simulink model "Valve_SimScape"  (R2023a)
settings: Solver=VariableStepAuto  StartTime=0.0  StopTime=8  RelTol=1e-3  AbsTol=1e-3
libraries: fl_lib x5, nesl_utility x5, SimscapeFluids_lib x1, simulink x1
settings Model: Creator=xuluyu  LastModifiedBy=xuluyu
settings SolverCC: AutoScaleAbsTol=off  AlgebraicLoopSolver=TrustRegion  MaxZcPerStep=1
settings DebuggingCC: UnconnectedInputMsg=warning  UnconnectedOutputMsg=warning  UnconnectedLineMsg=warning  SymbolicDimsDataTypeCodeGenerationDiagnostic=none
settings ModelReferenceCC: EnableRefExpFcnMdlSchedulingChecks=on
settings SFSimCC: CustomCodeUndefinedFunction=UseInterfaceOnly
settings RTWCC: DLArmComputeVersion=19.05
settings SimscapeCC: SimscapeLogType=all  SimscapeLogSimulationStatistics=on  SimscapeLogOpenViewer=on  SimscapeLogLimitData=off  SimscapeLogDataHistory=10000

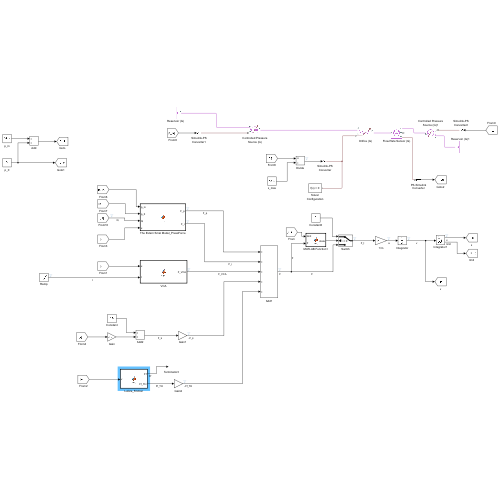
[thumbnail: Simulink's stored preview of the top-level diagram]
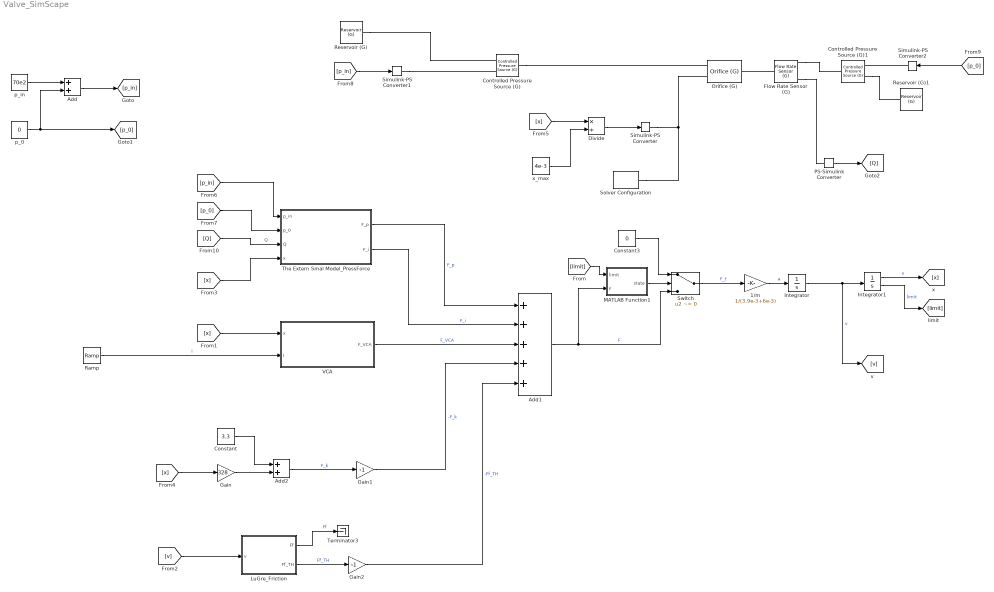
== system Valve_SimScape ==
  1/m : Gain  Gain=1/(3.9e-3+6e-3)
  Add : Sum
  Add1 : Sum  Inputs=+++++
  Add2 : Sum
  Constant : Constant  Value=3.3
  Constant3 : Constant  Value=0
  Controlled Pressure Source (G) : fl_lib/Gas/Sources/Controlled Pressure Source (G)  power_spec=foundation.enum.power_spec.isentropic  area_A=0.01 m^2  area_B=0.01 m^2
      settings: InternalSimscapePortConfiguration="{\"Bottom\":[],\"Left\":[{\"id\":\"A\",\"label\":\"A\",\"type\":\"foundation.gas.gas\"},{\"id\":\"P\",\"label\":\"P\",\"type\":\"input\"}],\"Right\":[{\"id\":\"B\",\"label\":\"B\",\"type\":\"foundation.gas.gas\"}],\"Top\":[]}"
  Controlled Pressure Source (G)1 : fl_lib/Gas/Sources/Controlled Pressure Source (G)  power_spec=foundation.enum.power_spec.isentropic  area_A=0.01 m^2  area_B=0.01 m^2
      settings: InternalSimscapePortConfiguration="{\"Bottom\":[],\"Left\":[{\"id\":\"A\",\"label\":\"A\",\"type\":\"foundation.gas.gas\"},{\"id\":\"P\",\"label\":\"P\",\"type\":\"input\"}],\"Right\":[{\"id\":\"B\",\"label\":\"B\",\"type\":\"foundation.gas.gas\"}],\"Top\":[]}"
  Divide : Product  Inputs=*/
  Flow Rate Sensor (G) : fl_lib/Gas/Sensors/Flow Rate Sensor (G)  mass_flow_measure=true  volumetric_flow_measure=true  volumetric_flow_conditions=foundation.enum.volumetric_flow_conditions.actual  p_std=0.101325 MPa  T_std=20 degC  energy_flow_measure=false
      settings: InternalSimscapePortConfiguration="{\"Bottom\":[],\"Left\":[{\"id\":\"A\",\"label\":\"A\",\"type\":\"foundation.gas.gas\"}],\"Right\":[{\"id\":\"B\",\"label\":\"B\",\"type\":\"foundation.gas.gas\"},{\"id\":\"M\",\"label\":\"M\",\"type\":\"output\"},{\"id\":\"V\",\"label\":\"V\",\"type\":\"output\"}],\"Top\":[]}"
  Gain : Gain  Gain=328
  Gain1 : Gain  Gain=-1
  Gain2 : Gain  Gain=-1
  Integrator : Integrator
  Integrator1 : Integrator  InitialCondition=1e-8  LimitOutput=on  UpperSaturationLimit=4e-3  LowerSaturationLimit=1e-8  ShowSaturationPort=on  ContinuousStateAttributes='x'
  LuGre_Friction : MATLAB Function  TreatAsAtomicUnit=on
  MATLAB Function1 : MATLAB Function  TreatAsAtomicUnit=on
  Orifice (G) : SimscapeFluids_lib/Gas/Valves & Orifices/Orifice (G)  orifice_type=foundation.enum.constant_variable.variable  orifice_parameterization=fluids.gas.valves_orifices.enum.OrificeParameterization.Cv  opening_characteristic=fluids.gas.valves_orifices.enum.OpeningCharacteristics.Tabulated  Cv_constant=4  Cv_max=4  L_Cv_TLU=Open_vector  Cv_TLU=Cv_valve  xT_Cv=0.7  Kv_constant=3.6  Kv_max=3.6  L_Kv_TLU=0 : 0.2 : 1  Kv_TLU=[1e-06, .72, 1.44, 2.16, 2.88, 3.6]  xT_Kv=0.7  C_constant=12 l/(bar*s)  B_crit_constant=0.3  C_max=12 l/(bar*s)  B_crit_linear=0.3  L_C_TLU=0 : 0.2 : 1  C_TLU=[1e-05, 2.4, 4.8, 7.2, 9.6, 12] l/(bar*s)  B_crit_TLU=0.3 * ones(1, 6)  m=0.5  T_ref_C=293.15 K  rho_ref_C=1.185 kg/m^3  orifice_area_constant=1e-4 m^2  orifice_area_max=1e-4 m^2  L_orifice_area_TLU=0 : 0.2 : 1  orifice_area_TLU=[1e-10, 2e-05, 4e-05, 6e-05, 8e-05, .0001] m^2  Cd=0.64  leakage_fraction=1e-6  smoothing_factor=0.01  B_lam=0.999  area=0.01 m^2
      settings: InternalSimscapePortConfiguration="{\"Bottom\":[],\"Left\":[{\"id\":\"A\",\"label\":\"A\",\"type\":\"foundation.gas.gas\"},{\"id\":\"L\",\"label\":\"L\",\"type\":\"input\"}],\"Right\":[{\"id\":\"B\",\"label\":\"B\",\"type\":\"foundation.gas.gas\"}],\"Top\":[]}"
  PS-Simulink Converter : nesl_utility/PS-Simulink Converter  PhysicalDomain=network_engine_domain  SubClassName=ps_output  LeftPortType=input  RightPortType=output  PseudoPeriodic=off  Frequencies=[]  VectorFormat=inherit  Unit=inherit  AffineConversion=off
  Ramp : simulink/Sources/Ramp  slope=1/5  start=1  InitialOutput=0
  Reservoir (G) : fl_lib/Gas/Elements/Reservoir (G)  pressure_spec=foundation.enum.pressure_spec.atmospheric  reservoir_pressure=0.101325 MPa  reservoir_temperature=293.15 K  area_A=0.01 m^2
  Reservoir (G)1 : fl_lib/Gas/Elements/Reservoir (G)  pressure_spec=foundation.enum.pressure_spec.atmospheric  reservoir_pressure=0.101325 MPa  reservoir_temperature=293.15 K  area_A=0.01 m^2
  Simulink-PS Converter : nesl_utility/Simulink-PS Converter  PhysicalDomain=network_engine_domain  SubClassName=ps_input  LeftPortType=input  RightPortType=output  PseudoPeriodic=off  Frequencies=[]  NoiseDistribution=none  NoiseParameters=[]  Unit=1  AffineConversion=off  FilteringAndDerivatives=provide  SimscapeFilterOrder=1  InputFilterTimeConstant=0.001  UdotUserProvided=0
  Simulink-PS Converter1 : nesl_utility/Simulink-PS Converter  PhysicalDomain=network_engine_domain  SubClassName=ps_input  LeftPortType=input  RightPortType=output  PseudoPeriodic=off  Frequencies=[]  NoiseDistribution=none  NoiseParameters=[]  Unit=Pa  AffineConversion=off  FilteringAndDerivatives=provide  SimscapeFilterOrder=1  InputFilterTimeConstant=0.001  UdotUserProvided=0
  Simulink-PS Converter2 : nesl_utility/Simulink-PS Converter  PhysicalDomain=network_engine_domain  SubClassName=ps_input  LeftPortType=input  RightPortType=output  PseudoPeriodic=off  Frequencies=[]  NoiseDistribution=none  NoiseParameters=[]  Unit=Pa  AffineConversion=off  FilteringAndDerivatives=provide  SimscapeFilterOrder=1  InputFilterTimeConstant=0.001  UdotUserProvided=0
  Solver Configuration : nesl_utility/Solver Configuration  PhysicalDomain=network_engine_domain  SubClassName=solver  LeftPortType=input  RightPortType=generic  Tones=[]  Harmonics=[]  SimulateNoise=off  Profile=off  UseLocalSampling=off  EnableSwitchedLinearOptims=on  FrequencyDomain=off  UseCCode=off  RelTol=0.001  AbsTol=1e-06  MinStep=1e-09  ToWorkspace=off  RevertToSquareIcSolve=off  NumHomotopyIterations=100  PhasorMode=off  PhasorModeNumHarmonics=1  ConsistencySolver=NEWTON_XTOL_AFTER_FTOL  IndexReductionMethod=DerivativeReplacement  DoDC=off  ResidualTolerance=1e-09  ConsistencyTolSource=GLOBAL  ConsistencyAbsTol=0.001  ConsistencyRelTol=0.001  ConsistencyTolFactor=0.001  UseLocalSolver=off  LocalSolverChoice=NE_BACKWARD_EULER_ADVANCER  ResolveIndetEquations=on  FunctionEvalNumThread=1  LocalSolverSampleTime=0.001  DoFixedCost=off  MaxNonlinIter=3  MaxModeIter=2  ComputeImpulses=off  ImpulseIterations=2  LinearAlgebra=auto  LinearAlgebraNumThread=0  EquationFormulation=NE_TIME_EF  DelaysMemoryBudget=1024  AutomaticFiltering=on  FilteringTimeConstant=0.001  PartitionStorageMethod=AS_NEEDED  PartitionMemoryBudget=1024  PartitionMethod=ROBUST
  Switch : Switch  Criteria=u2 ~= 0  SaturateOnIntegerOverflow=off  InputSameDT=off
  Terminator3 : Terminator
  The Extern Smal Model_PressForce : MATLAB Function  TreatAsAtomicUnit=on
  VCA : MATLAB Function  TreatAsAtomicUnit=on
  p_0 : Constant  Value=0
  p_in : Constant  Value=70e2
  x_max : Constant  Value=4e-3
  wires:
  [x] -> Gain/1
  Gain2/1 -> Add1/5  "-Ff_TH"
  MATLAB Function1/1(state) -> Switch/2
  Integrator1/1 -> [x]  "x"
  Switch/1 -> 1/m/1  "F_t"
  Add1/1 -> Switch/3, MATLAB Function1/2(F)  "F"
  1/m/1 -> Integrator/1  "a"
  Add2/1 -> Gain1/1  "F_k"
  The Extern Smal Model_PressForce/2(F_i) -> Add1/2  "F_i"
  Gain1/1 -> Add1/4  "-F_k"
  Integrator/1 -> [v], Integrator1/1  "v"
  LuGre_Friction/1(Ff) -> Terminator3/1  "Ff"
  Constant/1 -> Add2/1
  [limit] -> MATLAB Function1/1(limit)
  The Extern Smal Model_PressForce/1(F_p) -> Add1/1  "F_p"
  [v] -> LuGre_Friction/1(v)
  VCA/1(F_VCA) -> Add1/3  "F_VCA"
  [x] -> VCA/1(x)
  Constant3/1 -> Switch/1
  [x] -> The Extern Smal Model_PressForce/4(x)
  Integrator1/2 -> [limit]  "limit"
  LuGre_Friction/2(Ff_TH) -> Gain2/1  "Ff_TH"
  Gain/1 -> Add2/2
  [x] -> Divide/1
  x_max/1 -> Divide/2
  Divide/1 -> Simulink-PS Converter/1
  p_0/1 -> Add/2, [p_0]
  [p_in] -> The Extern Smal Model_PressForce/1(p_in)
  [p_0] -> The Extern Smal Model_PressForce/2(p_0)
  [p_in] -> Simulink-PS Converter1/1
  [p_0] -> Simulink-PS Converter2/1
  Add/1 -> [p_in]
  p_in/1 -> Add/1
  PS-Simulink Converter/1 -> [Q]
  [Q] -> The Extern Smal Model_PressForce/3(Q)  "Q"
  Ramp/1 -> VCA/2(I)  "I"
  connections:
  Simulink-PS Converter/RConn1 -- Solver Configuration/RConn1 -- Orifice (G)/LConn2
  Controlled Pressure Source (G)/RConn1 -- Orifice (G)/LConn1
  Simulink-PS Converter1/RConn1 -- Controlled Pressure Source (G)/LConn2
  Simulink-PS Converter2/RConn1 -- Controlled Pressure Source (G)1/LConn2
  Reservoir (G)/LConn1 -- Controlled Pressure Source (G)/LConn1
  Controlled Pressure Source (G)1/LConn1 -- Reservoir (G)1/LConn1
  Flow Rate Sensor (G)/LConn1 -- Orifice (G)/RConn1
  Flow Rate Sensor (G)/RConn1 -- Controlled Pressure Source (G)1/RConn1
  Flow Rate Sensor (G)/RConn3 -- PS-Simulink Converter/LConn1

== matlab function Valve_SimScape/VCA ==
  data: x input; F_VCA output; I input
function F_VCA  = fcn(x, I)
% VCA
% 音圈电磁力模型
% Pg-气隙磁导
% 默认音圈的永磁铁为圆柱形式
mu_0 = pi*4e-7;%磁导率，N*A^-2
r1 = 12e-3;%极片半径，m
r2 = 20e-3;%外壳半径，m
h = 10e-3;%极片高度，m
%Ag = (r2-r1)*h;%气隙磁路横截面，m^2
Ag = 2*pi*(r2+r1)*h;%气隙面积，m^2
Lg = 2*pi*(r1+r2)/2;%气隙长度，m
Pg = mu_0*Ag/Lg;%气隙磁导,H/m
%  气隙外总泄露磁导-Ptl
Dp = r1*2;%极片直径，m
Dy = r2*2;%扼片直径，m
Dm = 10e-3*2;%磁铁直径，m
Lm = 10e-3;%磁铁长度，m
Pf1 = 0.264*pi*mu_0*(Dp+Lg);
Pf2 = mu_0*(Dp+Lg)*log(1+Dp/Lg);
Pf3 = mu_0*(Dp+Lg)*log(1+(Dp-Dm)/Lg);
Pi = pi*mu_0*Lm*(Dm+Dy)/(4*(Dy-Dm));
Pl = pi*mu_0*sqrt(Dm*Lm/2);
P_ex = max(Pi,Pl);
Ptl = Pf1+Pf2+Pf3+P_ex;%气隙外总泄露磁导
% 磁导泄露系数-sigma
Pt = Pg+Ptl;%电路的总磁导
sigma = Pt/Pg;%磁导泄露系数
% 实际磁导-Pc
Am = 2*pi*(Dm/2)^2+2*pi*(Dm/2)*Lm;%磁铁面积，m^2
Pc = mu_0*(Ag*Lm/(Am*Lg))*sigma;
% 工作点的磁通密度-Bd
Br = 20;%最大磁通密度，H，不确定
mu_rec = 1*mu_0;%相对磁导率，不确定
Bd = Br/(1+mu_rec/Pc);
% 气隙的磁通密度-Bg
Bg = Am*Bd/(Ag*sigma);%气隙的磁通密度
% 气隙外磁通密度的归一化函数-Bnorm
ks = 20;%优化参数，针对不同的音圈需要调整
Bnorm = Lg/(ks*pi*x+Lg);
% 气隙上下的磁通密度-Ba,Bb
Ba = Bg*Bnorm;
Bb = Ba;
% 电磁力系数-Bl
% x_det_max = 9e-3;%线圈最大位移，m
% x_init = 0e-3;%线圈初始位移，m
xi = 5e-3;%内部线圈长度，m，小于Lm
xg = h/2;%气隙线圈长度，m
xo = 10e-4;%外部线圈长度，m
Number_Of_CoilTurns = 10e3;% 线圈匝数
% length_of_coil = 2e-3;% 线圈宽度，m
li = (xi-x)*2*pi*r1;
lg = xg*2*pi*r1;
lo = (xo+x)*2*pi*r1;
B_li = Bg*Lg*log(Lg+pi*ks*li)/(ks*pi)-Bg*Lg*log(Lg+pi*ks*0)/(ks*pi);
B_lg = Bg*lg;
B_lo = Bg*Lg*log(Lg+pi*ks*lo)/(ks*pi)-Bg*Lg*log(Lg+pi*ks*0)/(ks*pi);
B_t = (B_li+B_lg+B_lo)*Number_Of_CoilTurns;
% 电磁力-F
% I = 1;%线圈电流，A
F_VCA = B_t * I;
end

== matlab function Valve_SimScape/The Extern Smal Model_PressForce ==
  data: p_in input; p_0 input; Q input; x input; F_p output; F_i output
function [F_p,F_i] = fcn(p_in,p_0,Q,x)
% The Extended Smal Model
% 拓展的smal模型，包括流量模型、压力模型
% 阀座和膜片的几何参数
r_vi= 5e-3;%阀内进气腔半径，m
r_in = 5e-3;%阀外进气口半径，m
r_c = 6e-3;%阀内进气腔末端半径，m
r_m = 2e-3;%膜片半径，m
r_ex = 5e-3;%阀外出气口半径，m
% 流量模型-Flow Medel
zeta_in = 1-(r_vi/r_in)^4;%阀进气口的压力损失因子，1
zeta_ex = 1-(r_ex/r_c)^4;%阀出气口的压力损失因子，1
% x_det_max = 5e-3;%线圈最大位移，m
yr = x/(2*r_vi);%
zeta_yr = -6.1*exp(-4.13*yr)+0.497*(yr.^(-1.29))+1;%压力调整系数 
mu_air = 1.7894e-5;%空气粘度系数，Pa*s
rho_air = 1.248;%空气密度，kg/m^3
% 拓展的smal压力模型
p_vi = p_in - zeta_in*(rho_air/2).*(Q./(pi*r_vi^2)).^2;%阀内进气腔压力，Pa
p_c = p_0 + zeta_ex*(rho_air/2).*(Q./(pi*r_ex^2)).^2;%阀内进气腔末端压力，Pa
% 压力分布模型
n_yr = -29*exp(-77.2*yr)+27.8*exp(-17.5*yr);%压力分布指数
p1 = p_vi+rho_air/2*(Q/(pi*(r_vi)^2)).^2;%膜片中心压力
p2 = p1-rho_air/2*(Q./(2*pi*r_vi*x)).^2;%进气腔与膜片的交界处的压力
% 压力模型-Press Force Model
% a1 = pi*r_vi^2/2;
% a2 = pi*r_vi^2/2+pi*(pi*r_c^3+2*r_vi^3-3*r_c*r_vi^2)/(3*(r_c-r_vi));
a1 = n_yr./(n_yr+2)*(pi*r_vi^2);
a2 = 2./(n_yr+2)*pi*r_vi^2+pi*(pi*r_c^3+2*r_in^3-3*r_c*r_in^2)/(3*(r_c-r_in));
a3 = -1*pi*(pi*r_c^3+2*r_vi^3-3*r_c*r_vi^2)/(3*(r_c-r_vi))+pi*r_m^2-pi*r_vi^2;
a4 = pi*r_m^2;
F_p = a1*p1+a2*p2+a3*p_c-a4*p_0;% 膜片所受压力
F_i = 2*rho_air*Q.^2/(pi*r_in^2);% 流量导致的惯性力
end

== matlab function Valve_SimScape/LuGre_Friction ==
  data: v input; Ff output; Ff_TH output
function [Ff,Ff_TH] = fcn(v)
% LuGre_Friction
% LuGre摩擦力模型
% Columb-库伦摩擦-Fc
mu_c = 0.10;%动摩擦系数
Fn = 1;%法向力,N
Fc = mu_c*Fn;%库伦摩擦,N
% Viscous-粘性摩擦-Fv
% deta_v = 17.9e-6;%粘性系数，N*m^2/s
deta_v = 8e-1;%粘性系数，N*m^2/s 8e-1
Fv = deta_v*v;
% brk-临界摩擦-Fbrk
mu_b = 0.15;%临界(静)摩擦系数
Fbrk = mu_b*Fn;%临界摩擦,N
% Stribeck-斯特里贝克摩擦-Fs
cv = 100;
Fs = (Fbrk-Fc)*exp(-1*cv*abs(v))*sign(v);
% 总摩擦力-Ff
Ff = Fc+Fv+Fs;
% 总摩擦力-Ff
v_TH = 1e-4;% 速度阈值，m/s
if(abs(v)<v_TH)
    Ff_TH = abs(v)*sign(v)*(Fc+(Fbrk-Fc)*exp(-1*cv*v_TH))/v_TH;
else
    Ff_TH = Fc+((Fbrk-Fc)*exp(-1*cv*abs(v))*sign(v))+Fv;
end
end

== matlab function Valve_SimScape/MATLAB Function1 ==
  data: limit input; state output; F input
function state = fcn(limit,F)
if(limit==1 && F>0)
    state = 1;
elseif(limit==-1 && F<0)
    state = -1;
else
    state = 0;
end
